simulink subsystem "KDE_Qauternion_Attitude_of_Body_in_Geodetic"  (R2022a)
settings: Solver=VariableStepAuto  StartTime=0.0  StopTime=10.0  RelTol=1e-3
settings Model: Creator=Andrew Radulovich  LastModifiedBy=Andrew Radulovich

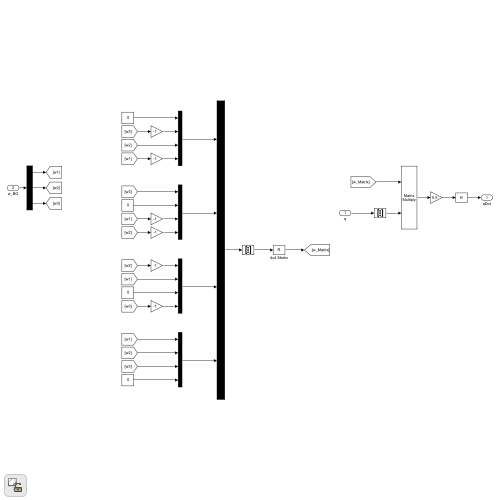
[thumbnail: Simulink's stored preview of the top-level diagram]
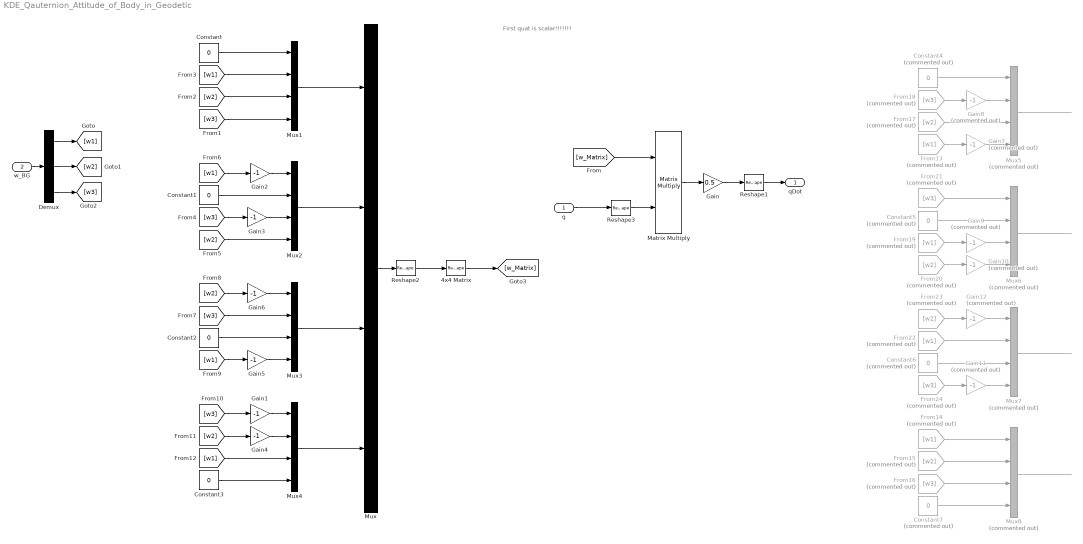
== system KDE_Qauternion_Attitude_of_Body_in_Geodetic ==
  note: First quat is scalar!!!!!!!
  q : Inport
  w_BG : Inport  Port=2
  4x4 Matrix : Reshape  OutputDimensionality=Customize  OutputDimensions=[4,4]
  Constant{,1..3} (4 alike) : Constant  Value=0
  Constant{4..7} (4 alike) : Constant  Commented=on  Value=0
  Demux : Demux  Outputs=3
  From{13..14,19,22} (4 alike) : From  Commented=on  GotoTag=w1
  From{15,17,20,23} (4 alike) : From  Commented=on  GotoTag=w2
  From{16,18,21,24} (4 alike) : From  Commented=on  GotoTag=w3
  Gain : Gain  Gain=0.5
  Gain{1..6} (6 alike) : Gain  Gain=-1
  Gain{7..12} (6 alike) : Gain  Commented=on  Gain=-1
  Matrix Multiply : Product  Multiplication=Matrix(*)
  Mux{,1..4} (5 alike) : Mux
  Mux{5..8} (4 alike) : Mux  Commented=on
  Reshape1 : Reshape  OutputDimensionality=Customize  OutputDimensions=[4,1]
  Reshape2 : Reshape  OutputDimensionality=Column vector (2-D)
  Reshape3 : Reshape  OutputDimensionality=Column vector (2-D)
  qDot : Outport
  wires:
  q/1 -> Reshape3/1
  Matrix Multiply/1 -> Gain/1
  w_BG/1 -> Demux/1
  Demux/1 -> [w1]
  Demux/2 -> [w2]
  Demux/3 -> [w3]
  [w_Matrix] -> Matrix Multiply/1
  Mux/1 -> Reshape2/1
  4x4 Matrix/1 -> [w_Matrix]
  Mux1/1 -> Mux/1
  Constant/1 -> Mux1/1
  [w3] -> Mux1/4
  Reshape2/1 -> 4x4 Matrix/1
  [w2] -> Mux1/3
  [w1] -> Mux1/2
  Mux2/1 -> Mux/2
  [w3] -> Gain3/1
  Mux3/1 -> Mux/3
  Mux4/1 -> Mux/4
  Constant3/1 -> Mux4/4
  [w3] -> Gain1/1
  [w2] -> Gain4/1
  [w1] -> Mux4/3
  [w1] -> Gain2/1
  Constant1/1 -> Mux2/2
  Gain3/1 -> Mux2/3
  [w2] -> Mux2/4
  Constant2/1 -> Mux3/3
  [w2] -> Gain6/1
  Gain6/1 -> Mux3/1
  [w3] -> Mux3/2
  [w1] -> Gain5/1
  Gain5/1 -> Mux3/4
  Reshape3/1 -> Matrix Multiply/2
  Gain/1 -> Reshape1/1
  Reshape1/1 -> qDot/1
  Gain9/1 -> Mux6/3
  From23/1 -> Gain12/1
  From22/1 -> Mux7/2
  From18/1 -> Gain8/1
  Gain11/1 -> Mux7/4
  Gain12/1 -> Mux7/1
  From21/1 -> Mux6/1
  From14/1 -> Mux8/1
  From15/1 -> Mux8/2
  Constant7/1 -> Mux8/4
  From17/1 -> Mux5/3
  From16/1 -> Mux8/3
  Mux6/1 -> ?
  Gain7/1 -> Mux5/4
  From19/1 -> Gain9/1
  From20/1 -> Gain10/1
  Constant6/1 -> Mux7/3
  Constant4/1 -> Mux5/1
  Mux5/1 -> ?
  Gain8/1 -> Mux5/2
  Gain10/1 -> Mux6/4
  Constant5/1 -> Mux6/2
  Mux8/1 -> ?
  From24/1 -> Gain11/1
  Mux7/1 -> ?
  From13/1 -> Gain7/1
  Gain2/1 -> Mux2/1
  Gain1/1 -> Mux4/1
  Gain4/1 -> Mux4/2
